simulink model "ADC_LED_CAN"  (R2016b)
settings: Solver=FixedStepDiscrete  StartTime=0.0  StopTime=10.0  RelTol=1e-3  EnableMultiTasking=on
libraries: c2837xDlib x2, simulink x2, c280xlib x2, c2802xlib x1
settings Model: ExtModeTrigDuration=8  Creator=admin  LastModifiedBy=admin
settings OptimizationCC: DefaultUnderspecifiedDataType=single  MaxStackSize=512
settings DebuggingCC: ParameterTunabilityLossMsg=error
settings HardwareCC: ProdBitPerChar=16  ProdBitPerInt=16  ProdBitPerPointer=32  ProdBitPerSizeT=32  ProdBitPerPtrDiffT=32  ProdLargestAtomicInteger=Integer  ProdLargestAtomicFloat=None  ProdWordSize=16  ProdLongLongMode=on  ProdHWDeviceType=Texas Instruments->C2000
settings RTWCC: SystemTargetFile=ert.tlc  HardwareBoard=TI Delfino F2837xD  TLCOptions=-aInlineSetEventsForThisBaseRateFcn=TLC_FALSE -aSuppressMultiTaskScheduler=TLC_FALSE -aRateBasedStepFcn=1  TemplateMakefile=ert_default_tmf  Description=Embedded Coder  GenerateReport=on  Toolchain=Texas Instruments Code Composer Studio v6 (C2000)  IncludeHyperlinkInReport=on  LaunchReport=on  GenerateTraceInfo=on  GenerateTraceReport=on  GenerateTraceReportSl=on  GenerateTraceReportSf=on  GenerateTraceReportEml=on
settings CodeAppCC: ForceParamTrailComments=on  IgnoreCustomStorageClasses=off  OperatorAnnotations=on  SimulinkDataObjDesc=on  SFDataObjDesc=on  MATLABFcnDesc=on  InsertBlockDesc=on  MATLABSourceComments=on
settings ERTTargetCC: CodeReplacementLibrary=TI C28x

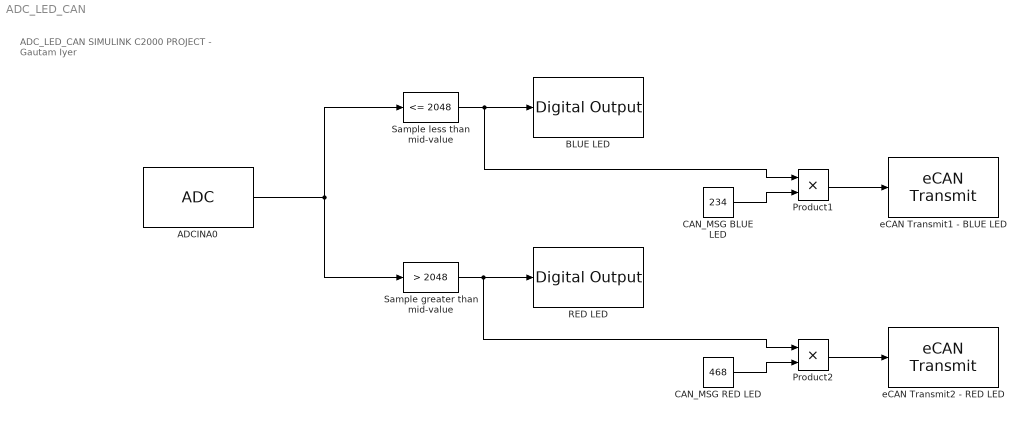
== system ADC_LED_CAN ==
  note: ADC_LED_CAN SIMULINK C2000 PROJECT
      |                                                    - Gautam Iyer
  ADCINA0 : c2802xlib/ADC  ADCModule=A  samplingMode=Single sample mode  ADCResolution=12-bit (Single-ended input)  useSOC1=SOC0  useSOC2=SOC0_SOC1  SOCAcquisitionWindow=7  SOCTriggerSource=CPU_TINT0n  SOCInterruptTrigger=No ADCINT  Ts=0.5  dType=uint16  postInterrupt=off  interruptSel=ADCINT1  ADCINTContinuous=on  endma=off  chdma=1  blkParamProc=C2000_Type4  conv1=ADCINA0  conv2=ADCINA0 and ADCINB0  conv1_Type4=ADCIN0  conv2_Type4=ADCIN0 and ADCIN1
  BLUE LED : c2837xDlib/Digital Output  GPIO_Number=GPIO24~GPIO31  GPIO_Bit0=off  GPIO_BIT0_Toggle=off  GPIO_Bit1=off  GPIO_BIT1_Toggle=off  GPIO_Bit2=off  GPIO_BIT2_Toggle=off  GPIO_Bit3=off  GPIO_BIT3_Toggle=off  GPIO_Bit4=off  GPIO_BIT4_Toggle=off  GPIO_Bit5=off  GPIO_BIT5_Toggle=off  GPIO_Bit6=off  GPIO_BIT6_Toggle=off  GPIO_Bit7=on  GPIO_BIT7_Toggle=on
  CAN_MSG BLUE LED : Constant  Value=234  OutDataTypeStr=uint32  SampleTime=0.5
  CAN_MSG RED LED : Constant  Value=468  OutDataTypeStr=uint32  SampleTime=0.5
  Product1 : Product  OutDataTypeStr=uint32
  Product2 : Product  OutDataTypeStr=uint32
  RED LED : c2837xDlib/Digital Output  GPIO_Number=GPIO32~GPIO39  GPIO_Bit0=off  GPIO_BIT0_Toggle=off  GPIO_Bit1=off  GPIO_BIT1_Toggle=off  GPIO_Bit2=on  GPIO_BIT2_Toggle=on  GPIO_Bit3=off  GPIO_BIT3_Toggle=off  GPIO_Bit4=off  GPIO_BIT4_Toggle=off  GPIO_Bit5=off  GPIO_BIT5_Toggle=off  GPIO_Bit6=off  GPIO_BIT6_Toggle=off  GPIO_Bit7=off  GPIO_BIT7_Toggle=off
  Sample greater than mid-value : simulink/Logic and Bit Operations/Compare To Constant  relop=>  const=2048  OutDataTypeStr=uint8
  Sample less than mid-value : simulink/Logic and Bit Operations/Compare To Constant  relop=<=  const=2048  OutDataTypeStr=uint8
  eCAN Transmit1 - BLUE LED : c280xlib/eCAN Transmit  chipFamily=C280x  useModule=eCAN_B  mailboxNo=0  messageID=12002345  messageType=Extended (29-bit identifier)  enableBlockingMode=on  postInterrupt=on  interruptLine=0
  "eCAN Transmit2 - RED LED " : c280xlib/eCAN Transmit  chipFamily=C280x  useModule=eCAN_B  mailboxNo=1  messageID=12002345  messageType=Extended (29-bit identifier)  enableBlockingMode=on  postInterrupt=on  interruptLine=0
  wires:
  ADCINA0/1 -> Sample less than mid-value/1, Sample greater than mid-value/1
  Sample less than mid-value/1 -> Product1/1, BLUE LED/1
  CAN_MSG BLUE LED/1 -> Product1/2
  Product1/1 -> eCAN Transmit1 - BLUE LED/1
  Sample greater than mid-value/1 -> Product2/1, RED LED/1
  CAN_MSG RED LED/1 -> Product2/2
  Product2/1 -> "eCAN Transmit2 - RED LED "/1
